simulink model "cable_test_ssc"  (R2015a)
settings: Solver=ode23t  StartTime=0.0  StopTime=50.0  RelTol=1e-3  AbsTol=1e-3
libraries: fl_lib x23, nesl_utility x3
settings Model: Creator=lkoelman  LastModifiedBy=lkoelman
settings SimscapeCC: SimscapeLogType=all  SimscapeLogDataHistory=10000

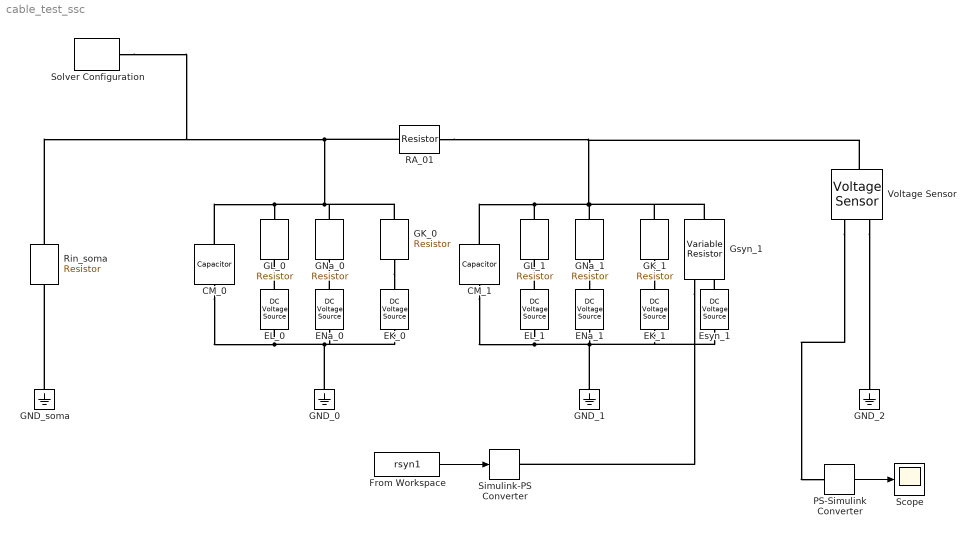
== system cable_test_ssc ==
  CM_0 : fl_lib/Electrical/Electrical Elements/Capacitor  c=1e-6 F  r=1e-6 Ohm  g=0 1/Ohm  i_specify=off  i_priority=High  i=0 A  v_specify=off  v_priority=High  v=0 V  vc_specify=off  vc_priority=High  vc=0 V
  CM_1 : fl_lib/Electrical/Electrical Elements/Capacitor  c=1e-6 F  r=1e-6 Ohm  g=0 1/Ohm  i_specify=off  i_priority=High  i=0 A  v_specify=off  v_priority=High  v=0 V  vc_specify=off  vc_priority=High  vc=0 V
  EK_0 : fl_lib/Electrical/Electrical Sources/DC Voltage Source  v0=-77 V
  EK_1 : fl_lib/Electrical/Electrical Sources/DC Voltage Source  v0=-77 V
  EL_0 : fl_lib/Electrical/Electrical Sources/DC Voltage Source  v0=-55 V
  EL_1 : fl_lib/Electrical/Electrical Sources/DC Voltage Source  v0=-55 V
  ENa_0 : fl_lib/Electrical/Electrical Sources/DC Voltage Source  v0=50 V
  ENa_1 : fl_lib/Electrical/Electrical Sources/DC Voltage Source  v0=50 V
  Esyn_1 : fl_lib/Electrical/Electrical Sources/DC Voltage Source  v0=70 V
  From Workspace : FromWorkspace  VariableName=rsyn1  SampleTime=0
  GK_0 : fl_lib/Electrical/Electrical Elements/Resistor  R=0.036 Ohm  i_specify=off  i_priority=High  i=0 A  v_specify=off  v_priority=High  v=0 V
  GK_1 : fl_lib/Electrical/Electrical Elements/Resistor  R=0.036 Ohm  i_specify=off  i_priority=High  i=0 A  v_specify=off  v_priority=High  v=0 V
  GL_0 : fl_lib/Electrical/Electrical Elements/Resistor  R=0.0003 Ohm  i_specify=off  i_priority=High  i=0 A  v_specify=off  v_priority=High  v=0 V
  GL_1 : fl_lib/Electrical/Electrical Elements/Resistor  R=0.0003 Ohm  i_specify=off  i_priority=High  i=0 A  v_specify=off  v_priority=High  v=0 V
  GND_0 : fl_lib/Electrical/Electrical Elements/Electrical Reference
  GND_1 : fl_lib/Electrical/Electrical Elements/Electrical Reference
  GND_2 : fl_lib/Electrical/Electrical Elements/Electrical Reference
  GND_soma : fl_lib/Electrical/Electrical Elements/Electrical Reference
  GNa_0 : fl_lib/Electrical/Electrical Elements/Resistor  R=0.12 Ohm  i_specify=off  i_priority=High  i=0 A  v_specify=off  v_priority=High  v=0 V
  GNa_1 : fl_lib/Electrical/Electrical Elements/Resistor  R=0.12 Ohm  i_specify=off  i_priority=High  i=0 A  v_specify=off  v_priority=High  v=0 V
  Gsyn_1 : fl_lib/Electrical/Electrical Elements/Variable Resistor  Rmin=0 Ohm  i_specify=off  i_priority=High  i=0 A  v_specify=off  v_priority=High  v=0 V
  PS-Simulink Converter : nesl_utility/PS-Simulink Converter  PhysicalDomain=network_engine_domain  SubClassName=ps_output  LeftPortType=input  RightPortType=output  PseudoPeriodic=off  Frequencies=[]  Unit=1  AffineConversion=off
  RA_01 : fl_lib/Electrical/Electrical Elements/Resistor  R=1 Ohm  i_specify=off  i_priority=High  i=0 A  v_specify=off  v_priority=High  v=0 V
  Rin_soma : fl_lib/Electrical/Electrical Elements/Resistor  R=1 Ohm  i_specify=off  i_priority=High  i=0 A  v_specify=off  v_priority=High  v=0 V
  Scope : Scope
  Simulink-PS Converter : nesl_utility/Simulink-PS Converter  PhysicalDomain=network_engine_domain  SubClassName=ps_input  LeftPortType=input  RightPortType=output  PseudoPeriodic=off  Frequencies=[]  NoiseDistribution=none  NoiseParameters=[]  Unit=1  AffineConversion=off  InputFiltering=off  SimscapeFilterOrder=1  InputFilterTimeConstant=0.001  UdotUserProvided=1
  Solver Configuration : nesl_utility/Solver Configuration  PhysicalDomain=network_engine_domain  SubClassName=solver  LeftPortType=input  RightPortType=generic  Accelerate=off  Tones=[]  Harmonics=[]  SimulateNoise=off  Profile=off  UseLocalSampling=off  EnableSwitchedLinearOptims=on  FrequencyDomain=off  UseCCode=off  RelTol=0.001  AbsTol=1e-06  MinStep=1e-09  ToWorkspace=off  RevertToSquareIcSolve=off  NumHomotopyIterations=100  DoDC=off  ResidualTolerance=1e-09  UseLocalSolver=off  LocalSolverChoice=NE_BACKWARD_EULER_ADVANCER  LocalSolverSampleTime=0.001  DoFixedCost=off  MaxNonlinIter=3  MaxModeIter=2  LinearAlgebra=Sparse  DelaysMemoryBudget=1024  AutomaticFiltering=on  FilteringTimeConstant=0.001
  Voltage Sensor : fl_lib/Electrical/Electrical Sensors/Voltage Sensor
  wires:
  PS-Simulink Converter/1 -> Scope/1
  From Workspace/1 -> Simulink-PS Converter/1
  connections:
  GL_0/RConn1 -- GK_0/RConn1 -- GNa_0/RConn1 -- Solver Configuration/RConn1 -- Rin_soma/RConn1 -- RA_01/LConn1 -- CM_0/RConn1
  EL_0/RConn1 -- EK_0/RConn1 -- ENa_0/RConn1 -- GND_0/LConn1 -- CM_0/LConn1
  ENa_0/LConn1 -- GNa_0/LConn1
  EL_0/LConn1 -- GL_0/LConn1
  CM_1/RConn1 -- Voltage Sensor/LConn1 -- RA_01/RConn1 -- GK_1/RConn1 -- Gsyn_1/RConn1 -- GNa_1/RConn1 -- GL_1/RConn1
  CM_1/LConn1 -- EK_1/RConn1 -- Esyn_1/RConn1 -- ENa_1/RConn1 -- GND_1/LConn1 -- EL_1/RConn1
  Esyn_1/LConn1 -- Gsyn_1/LConn2
  EL_1/LConn1 -- GL_1/LConn1
  GNa_1/LConn1 -- ENa_1/LConn1
  Gsyn_1/LConn1 -- Simulink-PS Converter/RConn1
  GND_soma/LConn1 -- Rin_soma/LConn1
  Voltage Sensor/RConn2 -- GND_2/LConn1
  Voltage Sensor/RConn1 -- PS-Simulink Converter/LConn1
  GK_0/LConn1 -- EK_0/LConn1
  GK_1/LConn1 -- EK_1/LConn1
